simulink subsystem "sensor_mag"  (R2026a)
settings: Solver=VariableStepAuto
model mask{samplingrate=100, noise_mag=[1,1,1]*1e-2, bias_mag=[0 0 0], scale_mag=[1 0 0; 0 1 0; 0 0 1], limit_mag=0, Ssi=[1 0 0; 0 1 0; 0 0 1], Lsi=[0 0 0], lon=80.5204, lat=43.4643, year=2025}
  mask prompts: samplingrate "Sampling Time (s)"; noise_mag "Mag Noise Power"; bias_mag "Mag Bias"; scale_mag "Mag Scaling"; limit_mag "Mag Limit"; Ssi "Body to Sensor rotation"; Lsi "Sensor Location in Body frame"; lon "Geodetic Longitude (deg)"; lat "Geodetic Latitude (deg)"; year "Year (decimal)"
undefined symbols (not defined in the file): location, WMM2025
libraries: simulink x1, aerolibgravity2 x1
settings Model: Creator=finnb  LastModifiedBy=trist

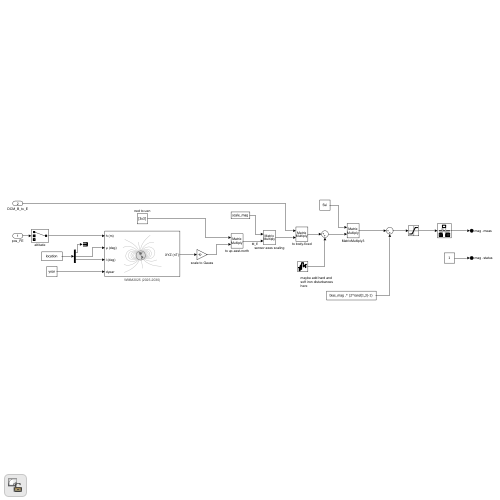
[thumbnail: Simulink's stored preview of the top-level diagram]
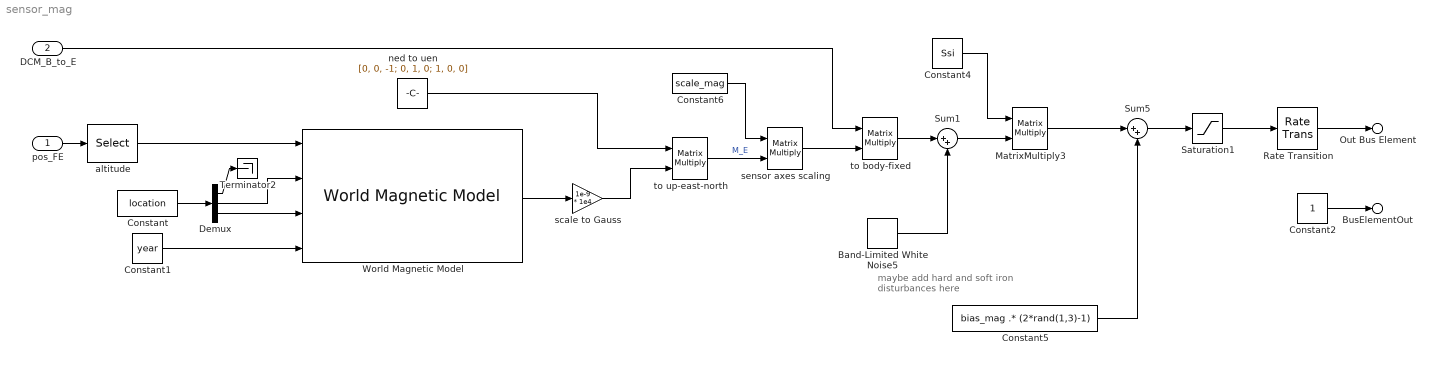
== system sensor_mag ==
  note: maybe add hard and soft iron disturbances here
  pos_FE : Inport
  DCM_B_to_E : Inport  Port=2
  Band-Limited White Noise5 : simulink/Sources/Band-Limited White Noise  Cov=noise_mag  Ts=samplingrate  seed=[298676]
  Constant : Constant  Value=location
  Constant1 : Constant  Value=year
  Constant2 : Constant  OutDataTypeStr=boolean
  Constant4 : Constant  Value=Ssi
  Constant5 : Constant  Value=bias_mag .* (2*rand(1,3)-1)
  Constant6 : Constant  Value=scale_mag
  Demux : Demux  Outputs=3
  MatrixMultiply3 : Product  Multiplication=Matrix(*)
  Rate Transition : RateTransition  OutPortSampleTime=samplingrate
  Saturation1 : Saturate  UpperLimit=limit_mag  LowerLimit=-limit_mag
  Sum1 : Sum  Inputs=|++
  Sum5 : Sum  Inputs=|++
  Terminator2 : Terminator
  World Magnetic Model : aerolibgravity2/World Magnetic Model  model=WMM2025 (2025-2030)  customFile='WMM2025.COF'  units=Metric (MKS)  time_in=on  month=January  day=1  year=2025  action=Error  h_out=off  dec_out=off  inc_out=off  ti_out=off
  altitude : Selector  InputPortWidth=3  IndexOptions=Index vector (dialog)  Indices=[1]  OutputSizes=1
  ned to uen : Constant  Value=[0, 0, -1; 0, 1, 0; 1, 0, 0]
  scale to Gauss : Gain  Gain=1e-9 * 1e4
  sensor axes scaling : Product  Multiplication=Matrix(*)
  to body-fixed : Product  Multiplication=Matrix(*)
  to up-east-north : Product  Multiplication=Matrix(*)
  Out Bus Element : Outport  PortName=mag  Element=meas
  BusElementOut : Outport  PortName=mag  Element=status
  wires:
  Constant/1 -> Demux/1
  Demux/2 -> World Magnetic Model/2
  World Magnetic Model/1 -> scale to Gauss/1
  to up-east-north/1 -> sensor axes scaling/2  "M_E"
  Band-Limited White Noise5/1 -> Sum1/2
  Sum1/1 -> MatrixMultiply3/2
  Constant4/1 -> MatrixMultiply3/1
  Demux/3 -> World Magnetic Model/3
  pos_FE/1 -> altitude/1
  Demux/1 -> Terminator2/1
  altitude/1 -> World Magnetic Model/1
  Constant1/1 -> World Magnetic Model/4
  to body-fixed/1 -> Sum1/1
  ned to uen/1 -> to up-east-north/1
  scale to Gauss/1 -> to up-east-north/2
  DCM_B_to_E/1 -> to body-fixed/1
  MatrixMultiply3/1 -> Sum5/1
  Sum5/1 -> Saturation1/1
  sensor axes scaling/1 -> to body-fixed/2
  Constant6/1 -> sensor axes scaling/1
  Saturation1/1 -> Rate Transition/1
  Rate Transition/1 -> Out Bus Element/1
  Constant2/1 -> BusElementOut/1
  Constant5/1 -> Sum5/2
